simulink model "Converter2_Boost"  (R2025a)
settings: Solver=ode15s  StartTime=0.0  StopTime=10  MaxStep=1e-4  RelTol=1e-4  EnableMultiTasking=on
libraries: spsCurrentMeasurementLib x5, spsSeriesRLCBranchLib x5, spsDCVoltageSourceLib x2, spsMosfetLib x2, spsVoltageMeasurementLib x2, spsControlledCurrentSourceLib x1, slpidlib x1, spsPWMGenerator2LevelLib x1, spsFirstOrderFilterLib x1, spsGroundLib x1, spspowerguiLib x1
settings Model: SimulationMode=accelerator  Creator=The MathWorks, Inc.  LastModifiedBy=kaust
settings SolverCC: MaxOrder=4.0  ZeroCrossAlgorithm=Adaptive  AlgebraicLoopSolver=TrustRegion
settings DataIOCC: LimitDataPoints=on  SaveFormat=Array  SaveOutput=off  SignalLogging=off  SaveTime=off  ReturnWorkspaceOutputs=off
settings OptimizationCC: ExpressionDepthLimit=2147483647.0  LifeSpan=inf
settings DebuggingCC: UnderspecifiedInitializationDetection=Classic  MergeDetectMultiDrivingBlocksExec=none  IgnoredZcDiagnostic=none  SolverPrmCheckMsg=warning  FcnCallInpInsideContextMsg=warning  UnconnectedInputMsg=warning  UnconnectedOutputMsg=warning  UnconnectedLineMsg=warning  StateNameClashWarn=warning  SFUnexpectedBacktrackingDiag=warning  SFNoUnconditionalDefaultTransitionDiag=warning  SFExecutionAtInitializationDiag=none  ArithmeticOperatorsInVariantConditions=warning
settings HardwareCC: ProdBitPerPointer=32.0  ProdBitPerSizeT=32.0  ProdBitPerPtrDiffT=32.0  ProdLargestAtomicFloat=None  ProdIntDivRoundTo=Undefined  ProdEndianess=Unspecified  ProdWordSize=32.0  ProdHWDeviceType=32-bit Generic
settings ModelReferenceCC: EnableRefExpFcnMdlSchedulingChecks=on  PropagateSignalLabelsOutOfModel=off
settings SFSimCC: SimUseLocalCustomCode=off  CustomCodeUndefinedFunction=UseInterfaceOnly
settings RTWCC: RTWUseLocalCustomCode=off  GPUComputeCapability=3.5  DLArmComputeVersion=19.05
settings CodeAppCC: StateflowObjectComments=on
settings GRTTargetCC: TargetLangStandard=C89/C90 (ANSI)  CombineOutputUpdateFcns=off  GRTInterface=on
settings ConfigComp: CovMetricSettings=dw  CovSaveCumulativeToWorkspaceVar=on  CovSaveSingleToWorkspaceVar=on  CovExternalEMLEnable=off  CovSFcnEnable=off
settings SimscapeCC: SimscapeNormalizeSystem=off  SimscapeNominalValues={1, 'bar'; 1, 'cm^3/s'; 1, 'bar*kg/s'; 1, 'kJ/kg'; 1, 'kW'; }

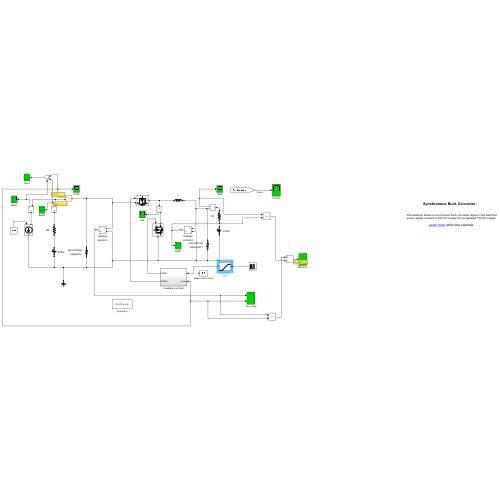
[thumbnail: Simulink's stored preview of the top-level diagram]
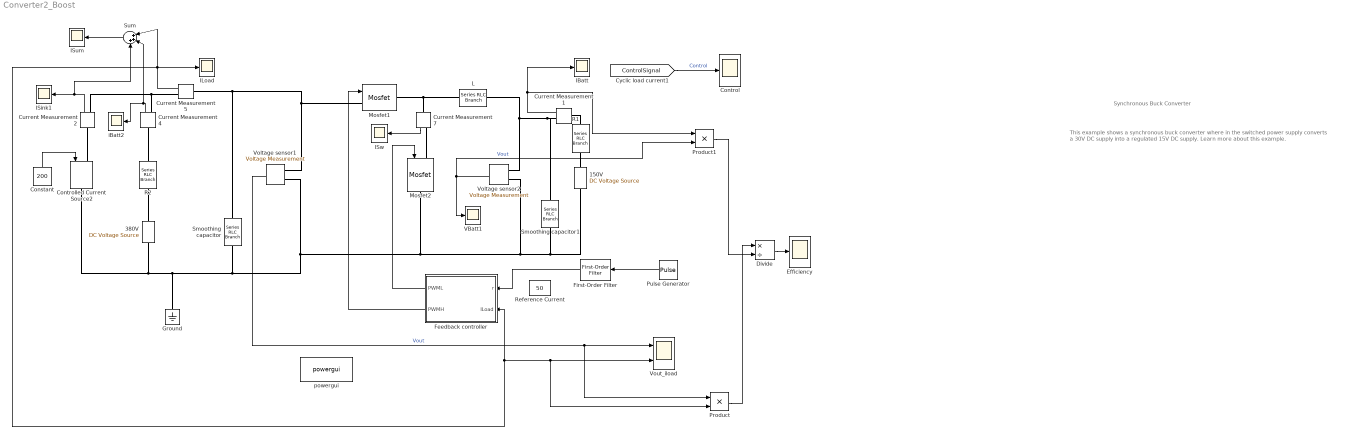
== system Converter2_Boost ==
  note: Synchronous Buck Converter
  note: This example shows a synchronous buck converter where in the switched power supply converts a 30V DC supply into a regulated 15V DC supply.
      |
      | Learn more about this example.
  150V : spsDCVoltageSourceLib/DC Voltage Source  Amplitude=150  Measurements=None
  380V : spsDCVoltageSourceLib/DC Voltage Source  Amplitude=380  Measurements=None
  Constant : Constant  Value=200
  Control : Scope
      settings: TimeSpan=0.01  ActiveDisplayYMinimum=-0.0024647053532001208  ActiveDisplayYMaximum=0.023182348178801094  DataLoggingVariableName=Control  DataLoggingSaveFormat=Array
  Controlled Current Source2 : spsControlledCurrentSourceLib/Controlled Current Source  Initialize=on  Source_Type=AC  Amplitude=0  Phase=0  Frequency=0  Measurements=None
  Current Measurement{1..2,4..5,7} (5 alike) : spsCurrentMeasurementLib/Current Measurement  PhasorSimulation=off  OutputType=Complex  PSBequivalent=0
  Divide : Product  Inputs=*/
  Efficiency : Scope
      settings: TimeSpan=0.01  ActiveDisplayYMinimum=-0.0024647053532001208  ActiveDisplayYMaximum=0.023182348178801094  DataLoggingVariableName=Control1  DataLoggingSaveFormat=Array
  Feedback controller : Subsystem
  First-Order Filter : spsFirstOrderFilterLib/First-Order Filter  FilterType=Lowpass  Tc=5e-3  Ts=0  Initialize=off  Vac_Init=[0, 0, 60]  Vdc_Init=0  PlotResponse=off  FreqRange="[0,  200,  1]"
  Ground : spsGroundLib/Ground  LConnTagsString=a
  IBatt : Scope
      settings: TimeSpan=0.01  ActiveDisplayYMinimum=-4410.7984256590225  ActiveDisplayYMaximum=16926.559366246598  DataLoggingVariableName=Isrc_sps1  DataLoggingSaveFormat=Array
  ILoad : Scope
      settings: TimeSpan=0.01  ActiveDisplayYMinimum=-119.68929460234355  ActiveDisplayYMaximum=1093.0850139818504  DataLoggingVariableName=Isrc_sps  DataLoggingSaveFormat=Array
  ISink1 : Scope
      settings: TimeSpan=0.01  ActiveDisplayYMinimum=-12.499999999999996  ActiveDisplayYMaximum=112.5  DataLoggingVariableName=Isrc_sps3  DataLoggingSaveFormat=Array
  ISum : Scope
      settings: TimeSpan=0.01  ActiveDisplayYMinimum=-1  ActiveDisplayYMaximum=1  DataLoggingVariableName=Isrc_sps4  DataLoggingSaveFormat=Array
  ISw : Scope
      settings: TimeSpan=0.01  ActiveDisplayYMinimum=-4410.7984256590225  ActiveDisplayYMaximum=16926.559366246598  DataLoggingVariableName=Isrc_sps6  DataLoggingSaveFormat=Array
  L : spsSeriesRLCBranchLib/Series RLC Branch  LConnTagsString=__new0  RConnTagsString=__new0  BranchType=L  Resistance=15  Inductance=1e-06  SetiL0=off  InitialCurrent=0  Capacitance=1e-6  Setx0=off  InitialVoltage=0  Measurements=None
  Mosfet1 : spsMosfetLib/Mosfet  Ron=0.1  Lon=0  Rd=0.01  Vfd=0.8  IC=0  Rs=1e5  Cs=inf  Measurements=off
  Mosfet2 : spsMosfetLib/Mosfet  Ron=0.1  Lon=0  Rd=0.01  Vfd=0.8  IC=0  Rs=1e4  Cs=inf  Measurements=off
  Product : Product
  Product1 : Product
  Pulse Generator : DiscretePulseGenerator  PulseType=Time based  Amplitude=50  Period=0.5  PulseWidth=50
  R1 : spsSeriesRLCBranchLib/Series RLC Branch  LConnTagsString=__new0  RConnTagsString=__new0  BranchType=R  Resistance=0.01  Inductance=1e-3  SetiL0=off  InitialCurrent=0  Capacitance=1e-6  Setx0=off  InitialVoltage=0  Measurements=None
  R2 : spsSeriesRLCBranchLib/Series RLC Branch  LConnTagsString=__new0  RConnTagsString=__new0  BranchType=R  Resistance=0.01  Inductance=1e-3  SetiL0=off  InitialCurrent=0  Capacitance=1e-6  Setx0=off  InitialVoltage=0  Measurements=None
  Reference Current : Constant  Value=50
  Smoothing capacitor : spsSeriesRLCBranchLib/Series RLC Branch  LConnTagsString=__new0  RConnTagsString=__new0  BranchType=C  Resistance=1  Inductance=1e-3  SetiL0=off  InitialCurrent=0  Capacitance=10e-3  Setx0=off  InitialVoltage=0  Measurements=None
  Smoothing capacitor1 : spsSeriesRLCBranchLib/Series RLC Branch  LConnTagsString=__new0  RConnTagsString=__new0  BranchType=C  Resistance=1  Inductance=1e-3  SetiL0=off  InitialCurrent=0  Capacitance=10e-3  Setx0=off  InitialVoltage=0  Measurements=None
  Sum : Sum  Inputs=|+++
  VBatt1 : Scope
      settings: TimeSpan=0.01  ActiveDisplayYMinimum=-4410.7984256590225  ActiveDisplayYMaximum=16926.559366246598  DataLoggingVariableName=Isrc_sps5  DataLoggingSaveFormat=Array
  Voltage sensor1 : spsVoltageMeasurementLib/Voltage Measurement  PhasorSimulation=off  OutputType=Complex  PSBequivalent=0
  Voltage sensor2 : spsVoltageMeasurementLib/Voltage Measurement  PhasorSimulation=off  OutputType=Complex  PSBequivalent=0
  Vout_iload : Scope  NumInputPorts=2
      settings: TimeSpan=0.01  ActiveDisplayYMinimum=377.75074454909316  ActiveDisplayYMaximum=380.24989171675594  DataLoggingVariableName=Vout_sps  DataLoggingSaveFormat=Array
  iBatt2 : Scope
      settings: TimeSpan=0.01  ActiveDisplayYMinimum=-12.499999999999996  ActiveDisplayYMaximum=112.5  DataLoggingVariableName=Isrc_sps2  DataLoggingSaveFormat=Array
  powergui : spspowerguiLib/powergui  Priority=1  SimulationMode=Continuous  SampleTime=50e-6  frequency=60  Iterations=50  frequencyindice=0  Pbase=100e6  ErrMax=1e-4  UnitsV=kV  UnitsW=MW  buscounter=0  FunctionMessages=off  echomessages=off  EnableUseOfTLC=off  CurrentSourceSwitches=off  DisableSnubberDevices=off  DisableRonSwitches=off  DisableVfSwitches=off  DisplayEquations=off  AutomaticDiscreteSolvers=off  SolverType=Tustin/Backward Euler (TBE)  Interpol=off  ExternalGateDelay=off  methode=off  Ts=100  x0status=blocks  SPID=on  SwTol=0  HookPort=off  NonlinearTolerance=1e-4  nMaxIteration=100  ContinueOnMaxIteration=off  RestoreLinks=warning  ResistiveCurrentMeasurement=off  Frange=[0:2:500]  Ylog=off  Xlog=on  ShowGrid=off  save=off  variable=ZData  structure=0  ZoomFFT=on  StartTime=0.0  cycles=1  DisplayStyle=1  fundamental=60  FreqAxis=off  MaxFrequency=1000  frequencyindicesteady=1  RmsSteady=1  display=off
  wires:
  Feedback controller/1(PWML) -> Mosfet2/1
  [ControlSignal] -> Control/1  "Control"
  Current Measurement5/1 -> Sum/1, ILoad/1, Feedback controller/2(ILoad), Product/2, Vout_iload/2
  Feedback controller/2(PWMH) -> Mosfet1/1
  Voltage sensor1/1 -> Product/1, Vout_iload/1  "Vout"
  Current Measurement1/1 -> IBatt/1, Product1/1
  Pulse Generator/1 -> First-Order Filter/1
  Constant/1 -> Controlled Current Source2/1
  Current Measurement4/1 -> iBatt2/1, Sum/2
  Current Measurement2/1 -> Sum/3, ISink1/1
  Sum/1 -> ISum/1
  Voltage sensor2/1 -> VBatt1/1, Product1/2  "Vout"
  Product/1 -> Divide/1
  Product1/1 -> Divide/2
  Divide/1 -> Efficiency/1
  Current Measurement7/1 -> ISw/1
  First-Order Filter/1 -> Feedback controller/1(r)
  connections:
  Mosfet2/RConn1 -- Smoothing capacitor/RConn1 -- Controlled Current Source2/RConn1 -- 380V/LConn1 -- Ground/LConn1 -- Voltage sensor1/LConn2 -- Smoothing capacitor1/RConn1 -- 150V/LConn1 -- Voltage sensor2/LConn2
  L/RConn1 -- Smoothing capacitor1/LConn1 -- Current Measurement1/RConn1 -- Voltage sensor2/LConn1
  L/LConn1 -- Current Measurement7/LConn1 -- Mosfet1/RConn1
  Smoothing capacitor/LConn1 -- Voltage sensor1/LConn1 -- Mosfet1/LConn1 -- Current Measurement5/LConn1
  150V/RConn1 -- R1/RConn1
  Current Measurement5/RConn1 -- Current Measurement2/RConn1 -- Current Measurement4/RConn1
  Current Measurement2/LConn1 -- Controlled Current Source2/LConn1
  380V/RConn1 -- R2/RConn1
  Current Measurement4/LConn1 -- R2/LConn1
  R1/LConn1 -- Current Measurement1/LConn1
  Current Measurement7/RConn1 -- Mosfet2/LConn1

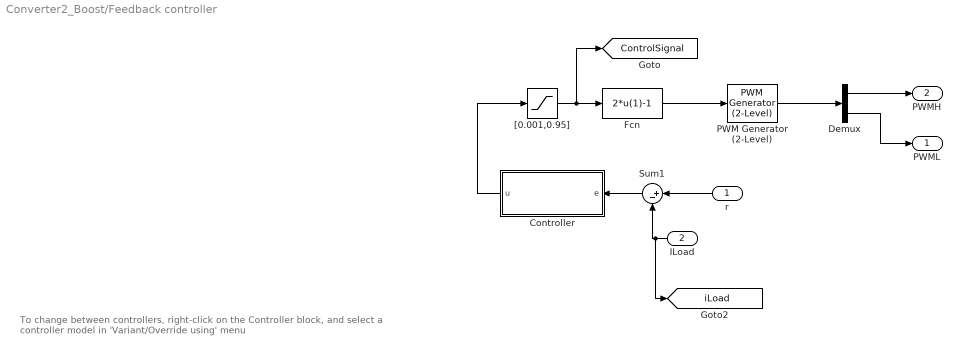
== system Converter2_Boost/Feedback controller ==
  note: To change between controllers, right-click on the Controller block,
      | and select a controller model in 'Variant/Override using' menu
  r : Inport
  ILoad : Inport  Port=2
  Controller : Subsystem  Variant=on  VariantControlMode=label  LabelModeActiveChoice=Variant1
      settings: AttributesFormatString=%<BlockChoice>
  Demux : Demux  Outputs=2
  Fcn : Fcn  Expr=2*u(1)-1
  PWM Generator (2-Level) : spsPWMGenerator2LevelLib/PWM Generator (2-Level)  ModulatorType=Single-phase half-bridge (2 pulses)  ModulatorMode=Unsynchronized  Fc=50000  Pc=90  nF=27  MinMax="[ -1  1 ]"  SamplingTechnique=Natural  ModulatingSignals=off  m=0.8  Freq=60  Phase=0  Ts=0  ShowCarrierOutport=off
  Sum1 : Sum  Inputs=|+-  InputSameDT=on  SaturateOnIntegerOverflow=on  OutDataTypeStr=Inherit: Same as first input
  "[0.001,0.95]" : Saturate  UpperLimit=0.95  LowerLimit=0.0001
  PWML : Outport  VectorParamsAs1DForOutWhenUnconnected=off
  PWMH : Outport  Port=2  VectorParamsAs1DForOutWhenUnconnected=off
  tag scope: ControlSignal=global, iLoad=global
  wires:
  Controller/1(u) -> "[0.001,0.95]"/1
  PWM Generator (2-Level)/1 -> Demux/1
  Demux/1 -> PWMH/1
  Demux/2 -> PWML/1
  Sum1/1 -> Controller/1(e)
  ILoad/1 -> [iLoad], Sum1/2
  "[0.001,0.95]"/1 -> [ControlSignal], Fcn/1
  r/1 -> Sum1/1
  Fcn/1 -> PWM Generator (2-Level)/1

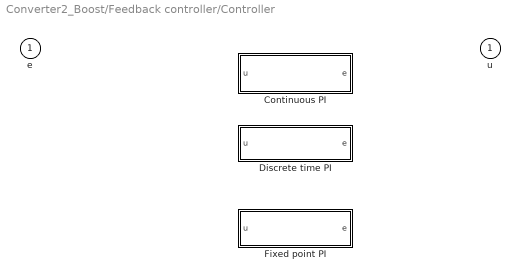
== system Converter2_Boost/Feedback controller/Controller ==
  e : Inport
  Continuous PI : Subsystem  VariantControl=Variant1
  Discrete time PI : Subsystem  VariantControl=Variant2
  Fixed point PI : Subsystem  MinMaxOverflowLogging=MinMaxAndOverflow  VariantControl=Variant3
  u : Outport  VectorParamsAs1DForOutWhenUnconnected=off

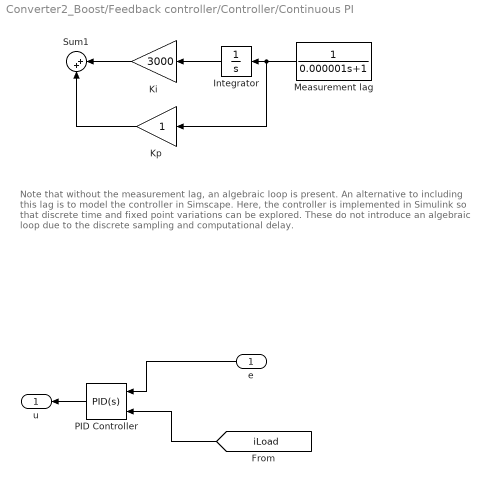
== system Converter2_Boost/Feedback controller/Controller/Continuous PI ==
  note: Note that without the measurement lag, an algebraic loop is present. An alternative to
      | including this lag is to model the controller in Simscape. Here, the controller is implemented
      | in Simulink so that discrete time and fixed point variations can be explored. These do not
      | introduce an algebraic loop due to the discrete sampling and computational delay.
  e : Inport
  Integrator : Integrator
  Ki : Gain  Gain=3000
  Kp : Gain
  Measurement lag : TransferFcn  Denominator=[0.000001 1]
  PID Controller : slpidlib/PID Controller  Controller=PID  Form=Parallel  TimeDomain=Continuous-time  UseExternalTs=off  SampleTime=-1  IntegratorMethod=Forward Euler  FilterMethod=Forward Euler  ControllerParametersSource=internal  P=0.01  I=1  UseKiTs=off  D=0.01  UseExternalDerivativeSource=off  N=100  UseFilter=on  TunerSelectOption=Transfer Function Based (PID Tuner App)  InitialConditionSource=internal  InitialConditionForIntegrator=0  InitialConditionForFilter=0  DifferentiatorICPrevScaledInput=0  ExternalReset=none  TrackingMode=on  Kt=0.01  LimitOutput=on  SatLimitsSource=internal  UpperSaturationLimit=1  LowerSaturationLimit=0  LinearizeAsGain=on  AntiWindupMode=back-calculation  Kb=0.05  LimitIntegrator=off  UpperIntegratorSaturationLimit=inf  LowerIntegratorSaturationLimit=-inf  POutMin=[]  POutMax=[]  IOutMin=[]  IOutMax=[]  DOutMin=[]  DOutMax=[]  NOutMin=[]  NOutMax=[]  SumOutMin=[]  SumOutMax=[]  SaturationOutMin=[]  SaturationOutMax=[]  PParamMin=[]  PParamMax=[]  IParamMin=[]  IParamMax=[]  DParamMin=[]  DParamMax=[]  NParamMin=[]  NParamMax=[]  KbParamMin=[]  KbParamMax=[]  KtParamMin=[]  KtParamMax=[]  KbOutMin=[]  KbOutMax=[]  KtOutMin=[]  KtOutMax=[]  IntegratorOutMin=[]  IntegratorOutMax=[]  FilterOutMin=[]  FilterOutMax=[]  SumI1OutMin=[]  SumI1OutMax=[]  SumI2OutMin=[]  SumI2OutMax=[]  SumI3OutMin=[]  SumI3OutMax=[]  SumI4OutMin=[]  SumI4OutMax=[]  SumDOutMin=[]  SumDOutMax=[]  DifferentiatorOutMin=[]  DifferentiatorOutMax=[]  FilterDiffOutCoefMin=[]  FilterDiffOutCoefMax=[]  ReciprocalOutMin=[]  ReciprocalOutMax=[]  SumDenOutMin=[]  SumDenOutMax=[]  SumNumOutMin=[]  SumNumOutMax=[]  DivideOutMin=[]  DivideOutMax=[]  UdiffTsProdOutMin=[]  UdiffTsProdOutMax=[]  NTsProdOutMin=[]  NTsProdOutMax=[]  UintegralTsProdOutMin=[]  UintegralTsProdOutMax=[]  UngainTsProdOutMin=[]  UngainTsProdOutMax=[]  ClampingZeroOutDataTypeStr=Inherit: Inherit via back propagation  ClampingZeroOutMin=[]  ClampingZeroOutMax=[]  FilterDenConstantOutDataTypeStr=Inherit: Inherit via back propagation  FilterDenConstantOutMin=[]  FilterDenConstantOutMax=[]  PCopyOutDataTypeStr=Inherit: Inherit via back propagation  PCopyOutMin=[]  PCopyOutMax=[]  NCopyOutDataTypeStr=Inherit: Inherit via back propagation  NCopyOutMin=[]  NCopyOutMax=[]  IntegratorContinuousStateAttributes=''  IntegratorStateMustResolveToSignalObject=off  IntegratorRTWStateStorageClass=Auto  FilterContinuousStateAttributes=''  FilterStateMustResolveToSignalObject=off  FilterRTWStateStorageClass=Auto  ParallelPVariant=InternalParameters  IdealPVariant=Disabled  IVariant=InternalParameters  DVariant=InternalParameters  IntegratorVariant=Continuous  SatVariant=Enabled  AWVariant=BackCalculation  PCopyVariant=Disabled  TRVariant=Enabled  FdbkBlocksVariant=Forward  IdealPFdbkVariant=Disabled  SatFdbkVariant=Disabled  DerivativeFilterVariant=ContFilter  NVariant=InternalParameters  NCopyVariant=Disabled  FilterICVariant=InternalICsFilter  IntegratorICVariant=InternalICs  ExternalResetVariant=Disabled  TRSumVariant=TrackingMode  SumFdbkVariant=Disabled  SumVariant=Sum_PID  TsampFilterVariant=InternalTs  TsampNgainVariant=Passthrough  TsampIntegralVariant=Disabled_SignalSpec  ExternalSaturationOutDataTypeStr=Inherit: Same as second input  DerivativeSourceVariant=ErrorSignal  PreIntVariant=InternalPreInt
  Sum1 : Sum  Inputs=|++  InputSameDT=on  SaturateOnIntegerOverflow=on  OutDataTypeStr=Inherit: Same as first input
  u : Outport  VectorParamsAs1DForOutWhenUnconnected=off
  wires:
  Measurement lag/1 -> Kp/1, Integrator/1
  Ki/1 -> Sum1/1
  Kp/1 -> Sum1/2
  Integrator/1 -> Ki/1
  [iLoad] -> PID Controller/2
  PID Controller/1 -> u/1
  e/1 -> PID Controller/1

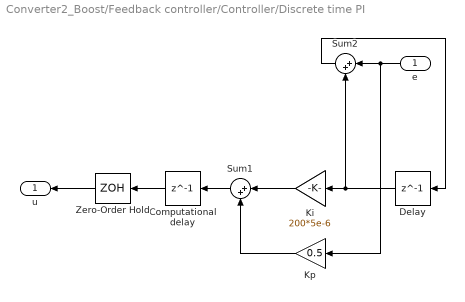
== system Converter2_Boost/Feedback controller/Controller/Discrete time PI ==
  e : Inport
  Computational delay : Delay  DelayLength=1  SampleTime=5e-6
  Delay : Delay  DelayLength=1  SampleTime=5e-6
  Ki : Gain  Gain=200*5e-6
  Kp : Gain  Gain=0.5
  Sum1 : Sum  Inputs=|++  InputSameDT=on  SaturateOnIntegerOverflow=on  OutDataTypeStr=Inherit: Same as first input
  Sum2 : Sum  Inputs=|++  InputSameDT=on  SaturateOnIntegerOverflow=on  OutDataTypeStr=Inherit: Same as first input
  Zero-Order Hold : ZeroOrderHold  SampleTime=5e-6
  u : Outport  VectorParamsAs1DForOutWhenUnconnected=off
  wires:
  Ki/1 -> Sum1/1
  Sum2/1 -> Delay/1
  Delay/1 -> Ki/1, Sum2/2
  Kp/1 -> Sum1/2
  Sum1/1 -> Computational delay/1
  e/1 -> Kp/1, Sum2/1
  Zero-Order Hold/1 -> u/1
  Computational delay/1 -> Zero-Order Hold/1

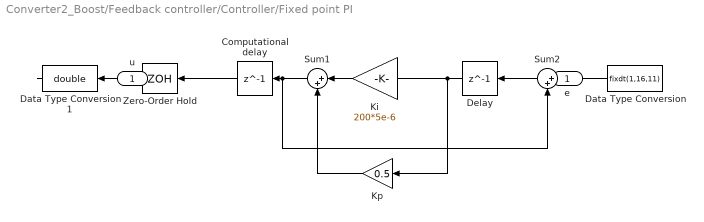
== system Converter2_Boost/Feedback controller/Controller/Fixed point PI ==
  e : Inport
  Computational delay : Delay  DelayLength=1  SampleTime=5e-6
  Data Type Conversion : DataTypeConversion  OutDataTypeStr=fixdt(1,16,11)  RndMeth=Nearest  SaturateOnIntegerOverflow=off
  Data Type Conversion1 : DataTypeConversion  OutDataTypeStr=double  RndMeth=Nearest  SaturateOnIntegerOverflow=off
  Delay : Delay  DelayLength=1  SampleTime=5e-6
  Ki : Gain  Gain=200*5e-6  OutDataTypeStr=fixdt(1,16,13)  RndMeth=Nearest
  Kp : Gain  Gain=0.5  OutDataTypeStr=fixdt(1,16,9)  RndMeth=Nearest
  Sum1 : Sum  Inputs=|++  SaturateOnIntegerOverflow=on
  Sum2 : Sum  Inputs=|++  InputSameDT=on  SaturateOnIntegerOverflow=on  OutDataTypeStr=Inherit: Same as first input
  Zero-Order Hold : ZeroOrderHold  SampleTime=5e-6
  u : Outport  VectorParamsAs1DForOutWhenUnconnected=off
  wires:
  Ki/1 -> Sum1/1
  Data Type Conversion1/1 -> u/1
  Data Type Conversion/1 -> Sum2/1, Kp/1
  Sum1/1 -> Computational delay/1
  Kp/1 -> Sum1/2
  e/1 -> Data Type Conversion/1
  Delay/1 -> Ki/1, Sum2/2
  Sum2/1 -> Delay/1
  Computational delay/1 -> Zero-Order Hold/1
  Zero-Order Hold/1 -> Data Type Conversion1/1
